simulink model "THEORETICAL_WAVEFORMS"  (R2016a)
settings: Solver=ode45  StartTime=0.0  StopTime=0.2  RelTol=1e-3
libraries: powerlib x19
settings Model: Creator=KARTHIK  LastModifiedBy=kalla
settings DataIOCC: SaveFormat=StructureWithTime
settings HardwareCC: ProdWordSize=32  ProdHWDeviceType=Specified

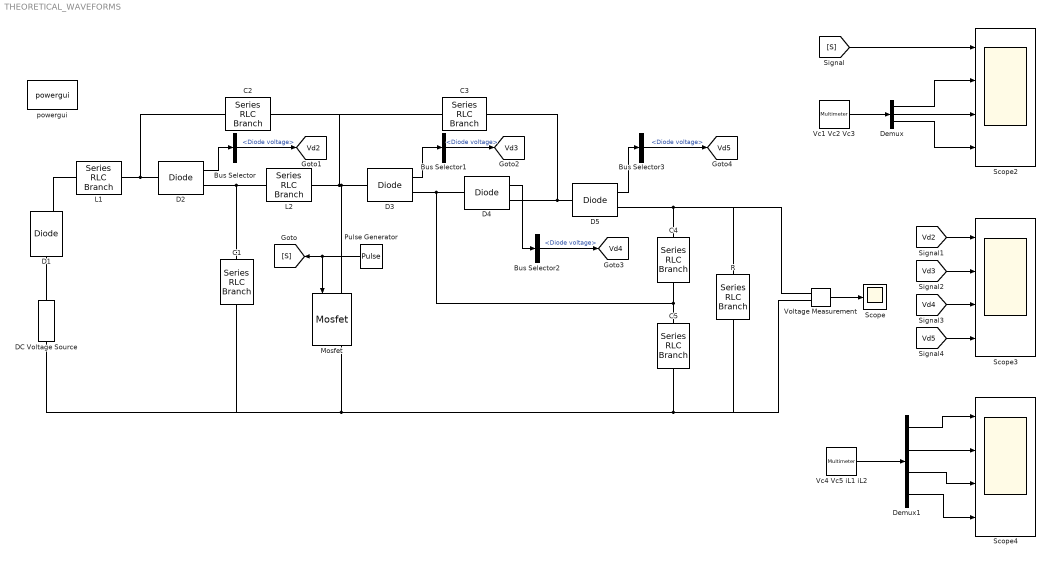
== system THEORETICAL_WAVEFORMS ==
  Bus Selector{,1..3} (4 alike) : BusSelector  OutputSignals=Diode voltage
  C{1,3..5} (4 alike) : powerlib/Elements/Series RLC Branch  LConnTagsString=__new0  RConnTagsString=__new0  BranchType=C  Resistance=1  Inductance=1e-3  SetiL0=off  InitialCurrent=0  Capacitance=520e-6  Setx0=off  InitialVoltage=0  Measurements=Branch voltage
  C2 : powerlib/Elements/Series RLC Branch  LConnTagsString=__new0  RConnTagsString=__new0  BranchType=C  Resistance=1  Inductance=1e-3  SetiL0=off  InitialCurrent=0  Capacitance=780e-6  Setx0=off  InitialVoltage=0  Measurements=Branch voltage
  D{1..5} (5 alike) : powerlib/Power Electronics/Diode  Ron=0.001  Lon=0  Vf=0.8  IC=0  UseSnubber=off  Rs=500  Cs=250e-9  Measurements=on
  DC Voltage Source : powerlib/Electrical Sources/DC Voltage Source  Amplitude=100  Measurements=None
  Demux : Demux  Outputs=3
  Demux1 : Demux
  L1 : powerlib/Elements/Series RLC Branch  LConnTagsString=__new0  RConnTagsString=__new0  BranchType=L  Resistance=1  Inductance=323e-6  SetiL0=off  InitialCurrent=0  Capacitance=1e-6  Setx0=off  InitialVoltage=0  Measurements=Branch current
  L2 : powerlib/Elements/Series RLC Branch  LConnTagsString=__new0  RConnTagsString=__new0  BranchType=L  Resistance=1  Inductance=318e-6  SetiL0=off  InitialCurrent=0  Capacitance=1e-6  Setx0=off  InitialVoltage=0  Measurements=Branch current
  Mosfet : powerlib/Power Electronics/Mosfet  Ron=0.1  Lon=0  Rd=0.01  Vfd=0  IC=0  Rs=1e5  Cs=inf  Measurements=on
  Pulse Generator : DiscretePulseGenerator  PulseType=Time based  Period=1/20e3  PulseWidth=26
  R : powerlib/Elements/Series RLC Branch  LConnTagsString=__new0  RConnTagsString=__new0  BranchType=R  Resistance=400  Inductance=1e-3  SetiL0=off  InitialCurrent=0  Capacitance=1e-6  Setx0=off  InitialVoltage=0  Measurements=None
  Scope : Scope
  Scope2 : Scope  NumInputPorts=4
  Scope3 : Scope  NumInputPorts=4
  Scope4 : Scope  NumInputPorts=4
  Vc1 Vc2 Vc3 : powerlib/Measurements/Multimeter  PhasorSimulation=off  OutputType=Complex  sel=[1 2 3]  L=7  Gain=[1 1 1]  yselected={'Ub: C1','Ub: C2','Ub: C3'};  PSBOutputType=1  PSBequivalent=0  AxesSetting=[0,0.1,-100,100]  Display=0  SavedBlockNames=-11
  Vc4 Vc5 iL1 iL2 : powerlib/Measurements/Multimeter  PhasorSimulation=off  OutputType=Complex  sel=[4 5 6 7]  L=7  Gain=[1 1 1 1]  yselected={'Ub: C4','Ub: C5','Ib: L1','Ib: L2'};  PSBOutputType=1  PSBequivalent=0  AxesSetting=[0,0.1,-100,100]  Display=0  SavedBlockNames=-11
  Voltage Measurement : powerlib/Measurements/Voltage Measurement  PhasorSimulation=off  OutputType=Complex  PSBequivalent=0
  powergui : powerlib/powergui  Priority=1  SimulationMode=Discrete  SolverType=Tustin  SampleTime=1e-7  frequency=60  SPID=off  DisableSnubberDevices=off  DisableRonSwitches=off  DisableVfSwitches=off  SwTol=0  DisplayEquations=off  Interpol=off  ExternalGateDelay=off  methode=off  Ts=10  FunctionMessages=off  echomessages=off  HookPort=off  EnableUseOfTLC=off  x0status=blocks  frequencyindice=0  Pbase=100e6  ErrMax=1e-4  Iterations=50  UnitsV=kV  UnitsW=MW  buscounter=0  RestoreLinks=warning  ResistiveCurrentMeasurement=off  Frange=[0:2:500]  Ylog=off  Xlog=on  ShowGrid=off  save=off  variable=ZData  structure=0  ZoomFFT=off  StartTime=0.0  cycles=1  DisplayStyle=1  fundamental=60  FreqAxis=off  MaxFrequency=1000  frequencyindicesteady=1  RmsSteady=1  display=off
  tag scope: Vd2=global, Vd3=global, Vd4=global, Vd5=global
  wires:
  Voltage Measurement/1 -> Scope/1
  [S] -> Scope2/1
  Vc1 Vc2 Vc3/1 -> Demux/1
  Demux/1 -> Scope2/2
  Demux/2 -> Scope2/3
  Demux/3 -> Scope2/4
  Vc4 Vc5 iL1 iL2/1 -> Demux1/1
  Demux1/1 -> Scope4/1
  Demux1/2 -> Scope4/2
  Demux1/3 -> Scope4/3
  Demux1/4 -> Scope4/4
  Bus Selector/1 -> [Vd2]  "<Diode voltage>"
  Bus Selector1/1 -> [Vd3]  "<Diode voltage>"
  D3/1 -> Bus Selector1/1
  D4/1 -> Bus Selector2/1
  Bus Selector2/1 -> [Vd4]  "<Diode voltage>"
  Bus Selector3/1 -> [Vd5]  "<Diode voltage>"
  D5/1 -> Bus Selector3/1
  [Vd2] -> Scope3/1
  [Vd3] -> Scope3/2
  [Vd4] -> Scope3/3
  [Vd5] -> Scope3/4
  Pulse Generator/1 -> [S], Mosfet/1
  D2/1 -> Bus Selector/1
  connections:
  L1/LConn1 -- D1/RConn1
  C2/RConn1 -- D2/LConn1 -- L1/RConn1
  L2/LConn1 -- C1/LConn1 -- D2/RConn1
  D3/LConn1 -- L2/RConn1 -- C3/RConn1 -- C2/LConn1 -- Mosfet/LConn1
  D4/RConn1 -- C3/LConn1 -- D5/LConn1
  D5/RConn1 -- R/LConn1 -- Voltage Measurement/LConn1 -- C4/LConn1
  DC Voltage Source/LConn1 -- C1/RConn1 -- Mosfet/RConn1 -- Voltage Measurement/LConn2 -- R/RConn1 -- C5/RConn1
  D4/LConn1 -- C4/RConn1 -- C5/LConn1 -- D3/RConn1
  D1/LConn1 -- DC Voltage Source/RConn1
